simulink model "BaselineController"  (Simulink 9.0)
settings: Solver=ode45  StartTime=0.0  StopTime=TMax  RelTol=1e-3  EnableMultiTasking=on
undefined symbols (not defined in the file or in its folder): alpha, DT, GenEff, OutList, PC_KI, PC_KK, PC_KP, PC_MaxPit, PC_MaxRat, PC_MinPit, PC_RefSpd, strmatch, VS_CtInSp, VS_MaxRat, VS_MaxTq, VS_Rgn2K, VS_RtPwr, VS_Slope15, VS_Slope25, VS_SySp
libraries: simulink x1
settings Model: Creator=Avell 1513  LastModifiedBy=Avell 1513
settings DataIOCC: LimitDataPoints=on
settings DebuggingCC: SolverPrmCheckMsg=warning  StateNameClashWarn=warning
settings GRTTargetCC: GeneratePreprocessorConditionals=Disable all

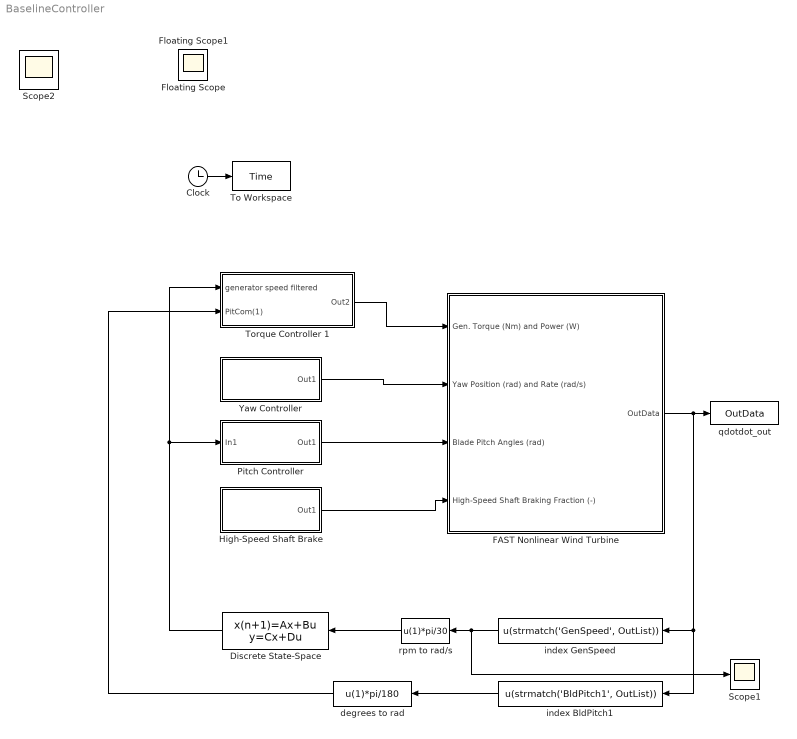
== system BaselineController ==
  Clock : Clock
  Discrete State-Space : DiscreteStateSpace  A=alpha  B=1-alpha  C=alpha  D=1-alpha  InitialCondition=122.40808744489746  SampleTime=DT
  FAST Nonlinear Wind Turbine : Subsystem  mask(FAST Nonlinear Wind Turbine){}
      mask help: This block contains the FAST S-Function.
      mask init:
      | clear FAST_SFunc
  High-Speed Shaft Brake : Subsystem
  Pitch Controller : Subsystem
  Scope1 : Scope
  To Workspace : ToWorkspace  VariableName=Time  SampleTime=-1
  Torque Controller 1 : Subsystem
  Yaw Controller : Subsystem
  degrees to rad : Fcn  Expr=u(1)*pi/180
  index BldPitch1 : Fcn  Expr=u(strmatch('BldPitch1', OutList))
  index GenSpeed : Fcn  Expr=u(strmatch('GenSpeed', OutList))
  qdotdot_out : ToWorkspace  VariableName=OutData  SampleTime=-1
  rpm to rad/s : Fcn  Expr=u(1)*pi/30  SampleTime=DT
  Floating Scope : Scope
  Floating Scope1 : Scope
  Scope2 : Scope
  wires:
  FAST Nonlinear Wind Turbine/1(OutData) -> index BldPitch1/1, index GenSpeed/1, qdotdot_out/1
  Yaw Controller/1(Out1) -> FAST Nonlinear Wind Turbine/2(Yaw Position (rad) and Rate (rad/s))
  Pitch Controller/1(Out1) -> FAST Nonlinear Wind Turbine/3(Blade Pitch Angles (rad))
  High-Speed Shaft Brake/1(Out1) -> FAST Nonlinear Wind Turbine/4(High-Speed Shaft Braking Fraction (-))
  index GenSpeed/1 -> rpm to rad/s/1, Scope1/1
  Clock/1 -> To Workspace/1
  index BldPitch1/1 -> degrees to rad/1
  degrees to rad/1 -> Torque Controller 1/2(PitCom(1))
  Torque Controller 1/1(Out2) -> FAST Nonlinear Wind Turbine/1(Gen. Torque (Nm) and Power (W))
  rpm to rad/s/1 -> Discrete State-Space/1
  Discrete State-Space/1 -> Pitch Controller/1(In1), Torque Controller 1/1(generator speed filtered)

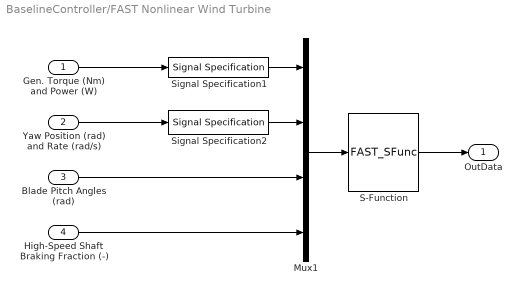
== system BaselineController/FAST Nonlinear Wind Turbine ==
  Gen. Torque (Nm) and Power (W) : Inport
  Yaw Position (rad) and Rate (rad/s) : Inport  Port=2
  Blade Pitch Angles (rad) : Inport  Port=3
  High-Speed Shaft Braking Fraction (-) : Inport  Port=4
  Mux1 : Mux
  S-Function : S-Function  FunctionName=FAST_SFunc  Parameters=FAST_InputFileName, TMax, 0  SFunctionDeploymentMode=off  EnableBusSupport=off
  Signal Specification1 : SignalSpecification  OutDataTypeStr=double  Dimensions=2
  Signal Specification2 : SignalSpecification  OutDataTypeStr=double  Dimensions=2
  OutData : Outport
  wires:
  Gen. Torque (Nm) and Power (W)/1 -> Signal Specification1/1
  S-Function/1 -> OutData/1
  Mux1/1 -> S-Function/1
  Blade Pitch Angles (rad)/1 -> Mux1/3
  Yaw Position (rad) and Rate (rad/s)/1 -> Signal Specification2/1
  Signal Specification1/1 -> Mux1/1
  Signal Specification2/1 -> Mux1/2
  High-Speed Shaft Braking Fraction (-)/1 -> Mux1/4

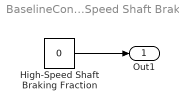
== system BaselineController/High-Speed Shaft Brake ==
  High-Speed Shaft Braking Fraction : Constant  Value=0
  Out1 : Outport
  wires:
  High-Speed Shaft Braking Fraction/1 -> Out1/1

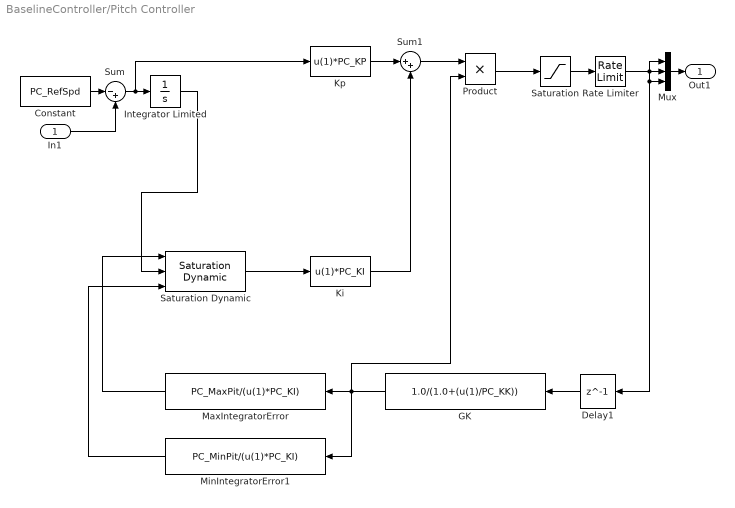
== system BaselineController/Pitch Controller ==
  In1 : Inport
  Constant : Constant  Value=PC_RefSpd
  Delay1 : Delay  DelayLength=1  InitialCondition=0  UseCircularBuffer=on  SampleTime=DT
  GK : Fcn  Expr=1.0/(1.0+(u(1)/PC_KK))
  Integrator Limited : Integrator  UpperSaturationLimit=PC_MaxPit  LowerSaturationLimit=PC_MinPit
  Ki : Fcn  Expr=u(1)*PC_KI
  Kp : Fcn  Expr=u(1)*PC_KP
  MaxIntegratorError : Fcn  Expr=PC_MaxPit/(u(1)*PC_KI)
  MinIntegratorError1 : Fcn  Expr=PC_MinPit/(u(1)*PC_KI)
  Mux : Mux  Inputs=3
  Product : Product
  Rate Limiter : RateLimiter  RisingSlewLimit=PC_MaxRat  FallingSlewLimit=-PC_MaxRat  SampleTimeMode=inherited
  Saturation : Saturate  UpperLimit=PC_MaxPit  LowerLimit=PC_MinPit
  Saturation Dynamic : simulink/Discontinuities/Saturation Dynamic  OutMin=[]  OutMax=[]  OutDataTypeStr=Inherit: Same as second input  OutDataType=fixdt(1, 16)  OutScaling=2^-10  DoSatur=off
  Sum : Sum  Inputs=|-+
  Sum1 : Sum  Inputs=|++
  Out1 : Outport
  wires:
  Sum/1 -> Kp/1, Integrator Limited/1
  Integrator Limited/1 -> Saturation Dynamic/2
  Kp/1 -> Sum1/1
  Saturation Dynamic/1 -> Ki/1
  Ki/1 -> Sum1/2
  Saturation/1 -> Rate Limiter/1
  Sum1/1 -> Product/1
  Product/1 -> Saturation/1
  Delay1/1 -> GK/1
  GK/1 -> MinIntegratorError1/1, Product/2, MaxIntegratorError/1
  Mux/1 -> Out1/1
  MaxIntegratorError/1 -> Saturation Dynamic/1
  MinIntegratorError1/1 -> Saturation Dynamic/3
  Rate Limiter/1 -> Mux/1, Mux/3, Delay1/1, Mux/2
  Constant/1 -> Sum/1
  In1/1 -> Sum/2

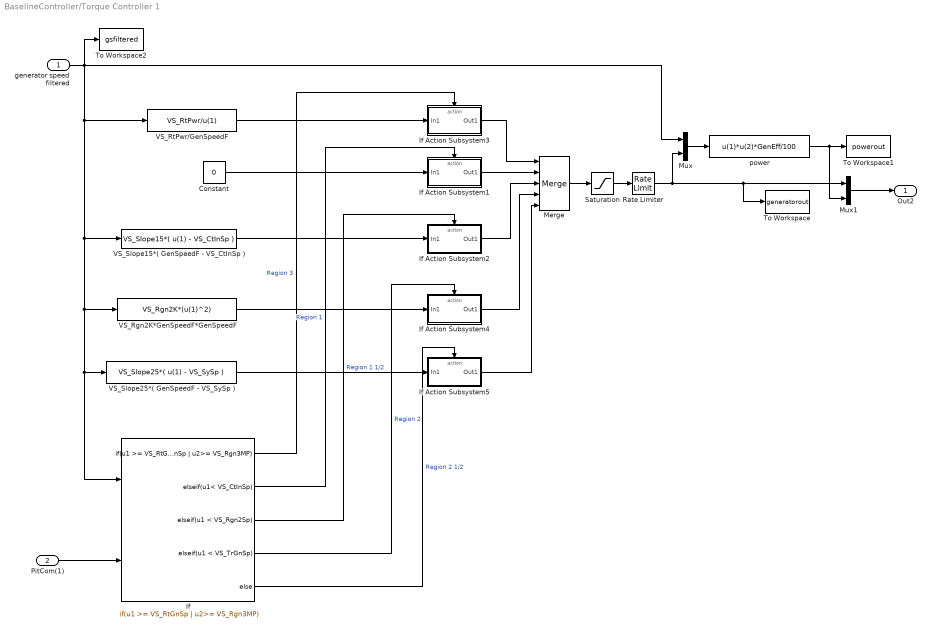
== system BaselineController/Torque Controller 1 ==
  generator speed filtered : Inport
  PitCom(1) : Inport  Port=2
  Constant : Constant  Value=0
  If : If  NumInputs=2  IfExpression=u1 >= VS_RtGnSp | u2>= VS_Rgn3MP  ElseIfExpressions=u1< VS_CtInSp, u1 < VS_Rgn2Sp, u1 < VS_TrGnSp
  If Action Subsystem1 : Subsystem  TreatAsAtomicUnit=on
  If Action Subsystem2 : Subsystem  TreatAsAtomicUnit=on
  If Action Subsystem3 : Subsystem  TreatAsAtomicUnit=on
  If Action Subsystem4 : Subsystem  TreatAsAtomicUnit=on
  If Action Subsystem5 : Subsystem  TreatAsAtomicUnit=on
  Merge : Merge  Inputs=5
  Mux : Mux  Inputs=2
  Mux1 : Mux  Inputs=2
  Rate Limiter : RateLimiter  RisingSlewLimit=VS_MaxRat  FallingSlewLimit=-VS_MaxRat  SampleTimeMode=inherited
  Saturation : Saturate  UpperLimit=VS_MaxTq  LowerLimit=0
  To Workspace : ToWorkspace  VariableName=generatorout  SampleTime=-1
  To Workspace1 : ToWorkspace  VariableName=powerout  SampleTime=-1
  To Workspace2 : ToWorkspace  VariableName=gsfiltered  SampleTime=-1
  VS_Rgn2K*GenSpeedF*GenSpeedF : Fcn  Expr=VS_Rgn2K*(u(1)^2)
  VS_RtPwr/GenSpeedF : Fcn  Expr=VS_RtPwr/u(1)
  VS_Slope15*( GenSpeedF - VS_CtInSp ) : Fcn  Expr=VS_Slope15*( u(1) - VS_CtInSp )
  VS_Slope25*( GenSpeedF - VS_SySp ) : Fcn  Expr=VS_Slope25*( u(1) - VS_SySp )
  power : Fcn  Expr=u(1)*u(2)*GenEff/100
  Out2 : Outport
  wires:
  If Action Subsystem2/1(Out1) -> Merge/3
  generator speed filtered/1 -> To Workspace2/1, Mux/1, If/1, VS_Slope25*( GenSpeedF - VS_SySp )/1, VS_Rgn2K*GenSpeedF*GenSpeedF/1, VS_Slope15*( GenSpeedF - VS_CtInSp )/1, VS_RtPwr/GenSpeedF/1
  If Action Subsystem1/1(Out1) -> Merge/2
  If Action Subsystem3/1(Out1) -> Merge/1
  If Action Subsystem4/1(Out1) -> Merge/4
  If/1 -> If Action Subsystem3/Action  "Region 3"
  VS_RtPwr/GenSpeedF/1 -> If Action Subsystem3/1(In1)
  If/2 -> If Action Subsystem1/Action  "Region 1"
  Constant/1 -> If Action Subsystem1/1(In1)
  If/3 -> If Action Subsystem2/Action  "Region 1 1/2"
  VS_Slope15*( GenSpeedF - VS_CtInSp )/1 -> If Action Subsystem2/1(In1)
  If/4 -> If Action Subsystem4/Action  "Region 2"
  VS_Rgn2K*GenSpeedF*GenSpeedF/1 -> If Action Subsystem4/1(In1)
  If/5 -> If Action Subsystem5/Action  "Region 2 1/2"
  If Action Subsystem5/1(Out1) -> Merge/5
  VS_Slope25*( GenSpeedF - VS_SySp )/1 -> If Action Subsystem5/1(In1)
  Merge/1 -> Saturation/1
  PitCom(1)/1 -> If/2
  Saturation/1 -> Rate Limiter/1
  Rate Limiter/1 -> To Workspace/1, Mux1/1, Mux/2
  Mux/1 -> power/1
  Mux1/1 -> Out2/1
  power/1 -> To Workspace1/1, Mux1/2

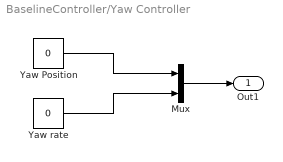
== system BaselineController/Yaw Controller ==
  Mux : Mux  Inputs=2
  Yaw Position : Constant  Value=0
  Yaw rate : Constant  Value=0
  Out1 : Outport
  wires:
  Mux/1 -> Out1/1
  Yaw Position/1 -> Mux/1
  Yaw rate/1 -> Mux/2

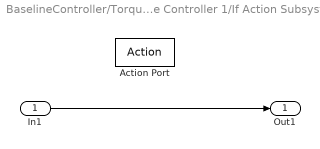
== system BaselineController/Torque Controller 1/If Action Subsystem1 ==
  In1 : Inport
  Action Port : ActionPort  ActionType=elseif
  Out1 : Outport
  wires:
  In1/1 -> Out1/1

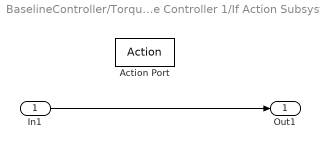
== system BaselineController/Torque Controller 1/If Action Subsystem2 ==
  In1 : Inport
  Action Port : ActionPort  ActionType=elseif
  Out1 : Outport
  wires:
  In1/1 -> Out1/1

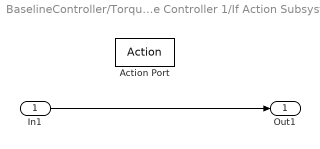
== system BaselineController/Torque Controller 1/If Action Subsystem3 ==
  In1 : Inport
  Action Port : ActionPort  ActionType=then
  Out1 : Outport
  wires:
  In1/1 -> Out1/1

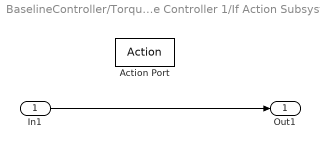
== system BaselineController/Torque Controller 1/If Action Subsystem4 ==
  In1 : Inport
  Action Port : ActionPort  ActionType=elseif
  Out1 : Outport
  wires:
  In1/1 -> Out1/1

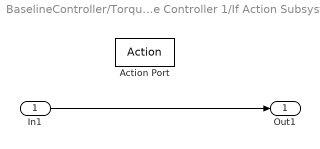
== system BaselineController/Torque Controller 1/If Action Subsystem5 ==
  In1 : Inport
  Action Port : ActionPort  ActionType=else
  Out1 : Outport
  wires:
  In1/1 -> Out1/1
